simulink model "grass"  (R2016b)
settings: Solver=VariableStepAuto  StartTime=0.0  StopTime=1000  RelTol=1e-3
undefined symbols (not defined in the file or in its folder): B, graze, qG, qU, Rg, Ru
settings Model: Creator=thomaskennedy  LastModifiedBy=thomaskennedy

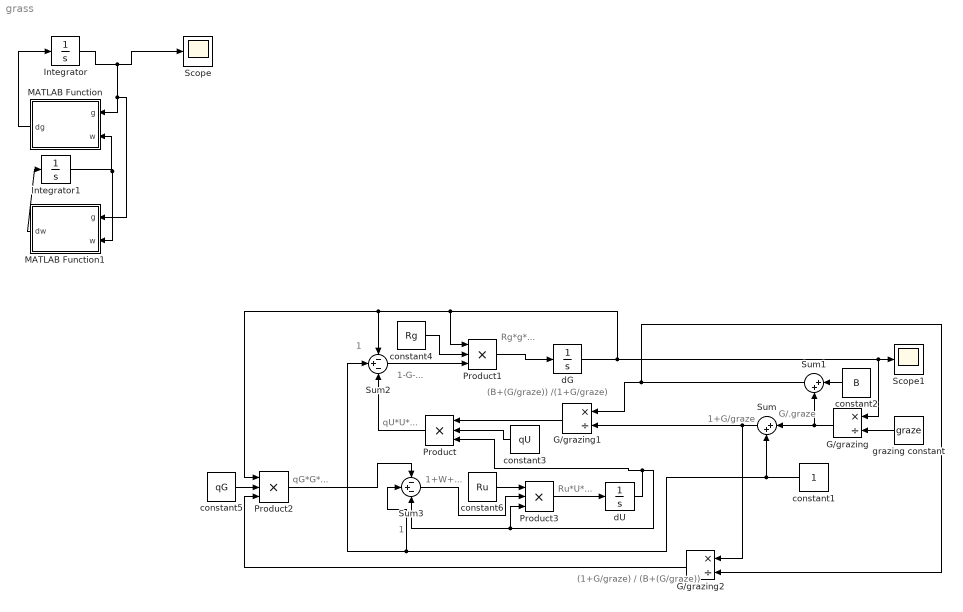
== system grass ==
  note: 1
  note: (B+(G/graze))
      | /(1+G/graze)
  note: 1+G/graze
  note: G/.graze
  note: 1
  note: (1+G/graze) /
      | (B+(G/graze))
  note: 1-G-...
  note: Rg*g*...
  note: qU*U*...
  note: qG*G*...
  note: 1+W+...
  note: Ru*U*...
  G/grazing : Product  Inputs=*/
  G/grazing1 : Product  Inputs=*/
  G/grazing2 : Product  Inputs=*/
  Integrator : Integrator  InitialCondition=.8
  Integrator1 : Integrator  InitialCondition=.2
  MATLAB Function : MATLAB Function  TreatAsAtomicUnit=on
  MATLAB Function1 : MATLAB Function  TreatAsAtomicUnit=on
  Product{,1..3} (4 alike) : Product  Inputs=3
  Scope : Scope
  Scope1 : Scope
  Sum : Sum  Inputs=|++
  Sum1 : Sum  Inputs=|++
  Sum2 : Sum  Inputs=-+-
  Sum3 : Sum  Inputs=-+-
  constant1 : Constant
  constant2 : Constant  Value=B
  constant3 : Constant  Value=qU
  constant4 : Constant  Value=Rg
  constant5 : Constant  Value=qG
  constant6 : Constant  Value=Ru
  dG : Integrator  InitialCondition=.8
  dU : Integrator  InitialCondition=.2
  grazing constant : Constant  Value=graze
  wires:
  Integrator/1 -> MATLAB Function1/1(g), MATLAB Function/1(g), Scope/1
  Integrator1/1 -> MATLAB Function/2(w), MATLAB Function1/2(w)
  MATLAB Function1/1(dw) -> Integrator1/1
  MATLAB Function/1(dg) -> Integrator/1
  grazing constant/1 -> G/grazing/2
  G/grazing/1 -> Sum/1, Sum1/2
  constant1/1 -> Sum2/2, Sum3/2, Sum/2
  Sum/1 -> G/grazing1/2, G/grazing2/1
  constant2/1 -> Sum1/1
  G/grazing1/1 -> Product/1
  dU/1 -> Product/3, Product3/3, Sum3/3
  constant3/1 -> Product/2
  Product/1 -> Sum2/3
  Sum2/1 -> Product1/3
  constant4/1 -> Product1/2
  Product1/1 -> dG/1
  Product2/1 -> Sum3/1
  Sum3/1 -> Product3/2
  constant6/1 -> Product3/1
  Product3/1 -> dU/1
  Sum1/1 -> G/grazing2/2, G/grazing1/1
  G/grazing2/1 -> Product2/3
  constant5/1 -> Product2/2
  dG/1 -> Product1/1, Sum2/1, Product2/1, Scope1/1, G/grazing/1

== matlab function grass/MATLAB Function1 ==
  data: g input; dw output; w input
function dw = fcn(g,w)
e=.492
dw = .4 * w * (1- w - 1.07*g*(1.0 + g/.492)/(.3+g/.492));

== matlab function grass/MATLAB Function ==
  data: g input; dg output; w input
function dg = fcn(g,w)
e=.492
dg = .27*g*(1-g-.6*w*(.3+(g/.492))/(1+g/.492));
